simulink model "station1_task"  (Simulink 3.00)
libraries: mathlib x3, candrvlib x1, logiclib x1, genlib x1

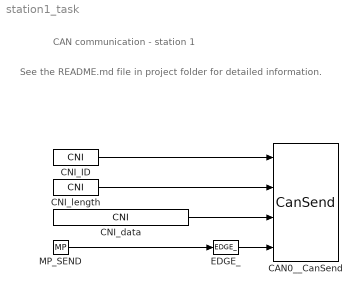
== system station1_task ==
  note: CAN communication - station 1
  note: See the README.md file in project folder for detailed information.
  CAN0__CanSend : candrvlib/CanSend  RTR=off  EXT=off
  CNI_ID : mathlib/CNI  icn=0x123
  CNI_data : mathlib/CNI  icn=0x87654321
  CNI_length : mathlib/CNI  icn=4
  EDGE_ : logiclib/EDGE_  iedge=1: Rising edge
  MP_SEND : genlib/MP  BSTATE=on  pwidth=1  RPTF=off
  wires:
  CNI_ID/1 -> CAN0__CanSend/1
  CNI_data/1 -> CAN0__CanSend/3
  CNI_length/1 -> CAN0__CanSend/2
  EDGE_/1 -> CAN0__CanSend/4
  MP_SEND/1 -> EDGE_/1
